simulink model "Suspension_system_nonlinear_dynamic_model"  (R2020a)
settings: Solver=FixedStepAuto  StartTime=0.0  StopTime=10  FixedStep=0.01  RelTol=1e-3
undefined symbols (not defined in the file): Ab1, Ab2, Agp, Ao1, Ao2, Apis, Ar, Arod, Av, b, Cdb1, Cdb2, Cdo1, Cdo2, Cdv1, Cdv2, Cf, Dpis, Dv1, Dv2, Fsp, k1, k2, l, Lg, mgp, Mpassm, mu, Pgasi, rho, slugs
libraries: simulink x9
settings Model: Creator=jmoyj  LastModifiedBy=jmoyj
settings DataIOCC: ReturnWorkspaceOutputs=off
settings DebuggingCC: ArithmeticOperatorsInVariantConditions=warning
settings SFSimCC: CustomCodeUndefinedFunction=UseInterfaceOnly

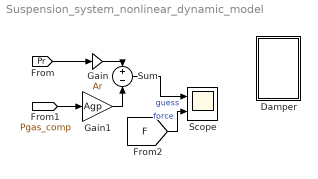
== system Suspension_system_nonlinear_dynamic_model ==
  Damper : Subsystem
  Gain : Gain  Gain=Ar
  Gain1 : Gain  Gain=Agp
  Scope : Scope  NumInputPorts=2
  Sum : Sum  Inputs=+-
  wires:
  [Pr] -> Gain/1
  [Pgas_comp] -> Gain1/1
  Gain/1 -> Sum/1
  Gain1/1 -> Sum/2
  Sum/1 -> Scope/1  "guess"
  [F] -> Scope/2  "force"

== system Suspension_system_nonlinear_dynamic_model/Damper ==
  Compression : Subsystem
  Final Values : Subsystem
  "Inputs_data " : Subsystem
  Rebound : Subsystem
  Scope10 : Scope
  Scope11 : Scope
  wires:
  "Inputs_data "/1(velocity) -> Scope11/1  "Velocity"
  "Inputs_data "/2(displacement) -> Scope10/1  "distance"

== system Suspension_system_nonlinear_dynamic_model/Damper/Compression ==
  " Q" : Subsystem
  CR : Subsystem
  CV : Subsystem
  Force : Subsystem
  Pgas and Pc : Subsystem
  Pr,Pc,Pv : Subsystem
  "Qb " : Subsystem
  Qlp : Subsystem
  "Qv " : Subsystem
  Scope : Scope  NumInputPorts=2
  Scope1 : Scope
  Sum : Sum  Inputs=|++
  "y " : Subsystem
  wires:
  [Pc_common] -> Sum/2, Scope/1
  [Pc_rebound] -> Sum/1, Scope/2
  Sum/1 -> Scope1/1

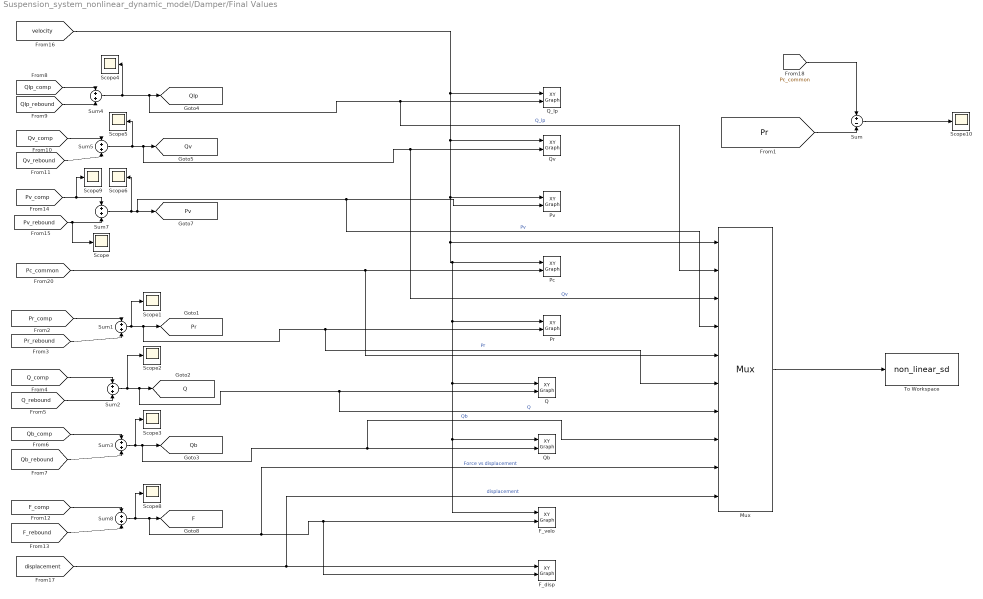
== system Suspension_system_nonlinear_dynamic_model/Damper/Final Values ==
  F_disp : simulink/Sinks/XY Graph  xmin=-1  xmax=+1  ymin=-20  ymax=30  st=-1
  F_velo : simulink/Sinks/XY Graph  xmin=-6  xmax=+6  ymin=-20  ymax=20  st=-1
  Mux : Mux  Inputs=10
  Pc : simulink/Sinks/XY Graph  xmin=-6  xmax=+6  ymin=20  ymax=30  st=-1
  Pr : simulink/Sinks/XY Graph  xmin=-6  xmax=+6  ymin=5  ymax=45  st=-1
  Pv : simulink/Sinks/XY Graph  xmin=-6  xmax=+6  ymin=12  ymax=40  st=-1
  Q : simulink/Sinks/XY Graph  xmin=-6  xmax=+6  ymin=0  ymax=5  st=-1
  Q_lp : simulink/Sinks/XY Graph  xmin=-6  xmax=6  ymin=0  ymax=0.005  st=-1
  Qb : simulink/Sinks/XY Graph  xmin=-6  xmax=+6  ymin=0  ymax=5  st=-1
  Qv : simulink/Sinks/XY Graph  xmin=-6  xmax=+6  ymin=0  ymax=1.5  st=-1
  Scope{,1..6,8..10} (10 alike) : Scope
  Sum : Sum  Inputs=+-
  Sum{1..5,7..8} (7 alike) : Sum
  To Workspace : ToWorkspace  VariableName=non_linear_sd  SaveFormat=Timeseries  SampleTime=-1
  tag scope: F=global, Pr=global, Pv=global, Q=global, Qb=global, Qlp=global, Qv=global
  wires:
  Sum1/1 -> Scope1/1, Mux/6, Pr/2, [Pr]  "Pr"
  [Pr_comp] -> Sum1/1
  [Pr_rebound] -> Sum1/2
  Sum2/1 -> Scope2/1, Mux/7, Q/2, [Q]  "Q"
  [Q_comp] -> Sum2/1
  [Q_rebound] -> Sum2/2
  Sum3/1 -> Scope3/1, Mux/8, Qb/2, [Qb]  "Qb"
  [Qb_comp] -> Sum3/1
  [Qb_rebound] -> Sum3/2
  Sum4/1 -> Scope4/1, Mux/2, Q_lp/2, [Qlp]  "Q_lp"
  [Qlp_comp] -> Sum4/1
  [Qlp_rebound] -> Sum4/2
  Sum5/1 -> Scope5/1, Mux/3, Qv/2, [Qv]  "Qv"
  [Qv_comp] -> Sum5/1
  [Qv_rebound] -> Sum5/2
  [Pv_rebound] -> Scope/1, Sum7/2
  Sum7/1 -> Scope6/1, Mux/4, Pv/2, [Pv]  "Pv"
  [Pv_comp] -> Scope9/1, Sum7/1
  Sum8/1 -> Scope8/1, Mux/9, F_disp/2, F_velo/2, [F]  "Force vs displacement"
  [F_comp] -> Sum8/1
  [F_rebound] -> Sum8/2
  [velocity] -> Mux/1, F_velo/1, Qb/1, Q/1, Pr/1, Pc/1, Pv/1, Qv/1, Q_lp/1
  [displacement] -> Mux/10, F_disp/1  "displacement"
  Mux/1 -> To Workspace/1
  [Pc_common] -> Sum/1
  [Pr] -> Sum/2
  Sum/1 -> Scope10/1
  [Pc_common] -> Mux/5, Pc/2

== system Suspension_system_nonlinear_dynamic_model/Damper/Inputs_data  ==
  Derivative : Derivative
  Derivative1 : Derivative
  Scope : Scope
  Scope1 : Scope
  Scope2 : Scope
  Sine Wave : Sin  Amplitude=0.499  Frequency=1.59*2*pi  Phase=-(pi/2)  SampleTime=0
  velocity : Outport  VectorParamsAs1DForOutWhenUnconnected=off
  displacement : Outport  Port=2  VectorParamsAs1DForOutWhenUnconnected=off
  tag scope: acceleration=global, displacement=global, velocity=global
  wires:
  Derivative1/1 -> [acceleration], Scope2/1
  Derivative/1 -> velocity/1, Scope1/1, [velocity], Derivative1/1
  Sine Wave/1 -> Derivative/1, displacement/1, Scope/1, [displacement]

== system Suspension_system_nonlinear_dynamic_model/Damper/Rebound ==
  " Q" : Subsystem
  Force Model : Subsystem
  Pc,Pr,Pv : Subsystem
  Pgas and Pc : Subsystem
  "Qb " : Subsystem
  Qlp : Subsystem
  "Qv " : Subsystem
  RC : Subsystem
  RV : Subsystem
  "y " : Subsystem

== system Suspension_system_nonlinear_dynamic_model/Damper/Compression/ Q ==
  Constant : Constant  Value=Ar
  Constant1 : Constant  Value=0
  Product : Product
  Scope : Scope
  Sign : Signum
  Switch : Switch  Criteria=u2 > Threshold
  tag scope: Q_comp=global
  wires:
  Constant/1 -> Product/2
  [velocity] -> Sign/1, Product/1
  Product/1 -> Switch/1
  Sign/1 -> Switch/2
  Constant1/1 -> Switch/3
  Switch/1 -> Scope/1, [Q_comp]

== system Suspension_system_nonlinear_dynamic_model/Damper/Compression/CR ==
  Constant : Constant  Value=rho
  Constant1 : Constant  Value=2
  Constant2 : Constant  Value=slugs
  Constant3 : Constant  Value=Ab1
  Constant4 : Constant  Value=Cdb1
  Delay : Delay  DelayLength=0  InitialCondition=0.02
  Product : Product
  Product1 : Product  Inputs=3
  Product2 : Product  Inputs=*/
  Product3 : Product
  Scope1 : Scope
  Scope2 : Scope
  Square : Math  Operator=square  SignedPower=on  SaturateOnIntegerOverflow=on
  Square1 : Math  Operator=square  SignedPower=on  SaturateOnIntegerOverflow=on
  tag scope: CR=global
  wires:
  Product1/1 -> Product2/2
  Product/1 -> Product2/1
  Square1/1 -> Product1/3
  Constant/1 -> Product/1
  Constant2/1 -> Product1/2
  Constant4/1 -> Product3/2
  Constant1/1 -> Product1/1
  Square/1 -> Product/2
  [Qb_comp] -> Scope1/1, Square/1
  Product3/1 -> Square1/1
  Constant3/1 -> Product3/1
  Product2/1 -> Scope2/1, Delay/1
  Delay/1 -> [CR]

== system Suspension_system_nonlinear_dynamic_model/Damper/Compression/CV ==
  Constant : Constant  Value=rho
  Constant1 : Constant  Value=2
  Constant2 : Constant  Value=slugs
  Constant3 : Constant  Value=Ao1
  Constant4 : Constant  Value=Cdo1
  Delay : Delay  DelayLength=0  InitialCondition=0.16
  Product : Product
  Product1 : Product  Inputs=3
  Product2 : Product  Inputs=*/
  Product3 : Product
  Scope{,1..3} (4 alike) : Scope
  Square : Math  Operator=square  SignedPower=on  SaturateOnIntegerOverflow=on
  Square1 : Math  Operator=square  SignedPower=on  SaturateOnIntegerOverflow=on
  tag scope: CV=global
  wires:
  Product1/1 -> Product2/2, Scope2/1
  Product/1 -> Product2/1
  Square1/1 -> Product1/3
  Constant/1 -> Product/1
  Constant2/1 -> Product1/2
  Constant4/1 -> Product3/2
  Constant1/1 -> Product1/1
  Square/1 -> Product/2
  [Qv_comp] -> Scope/1, Square/1
  Product3/1 -> Square1/1
  Constant3/1 -> Product3/1
  Delay/1 -> Scope3/1, [CV]
  Product2/1 -> Scope1/1, Delay/1

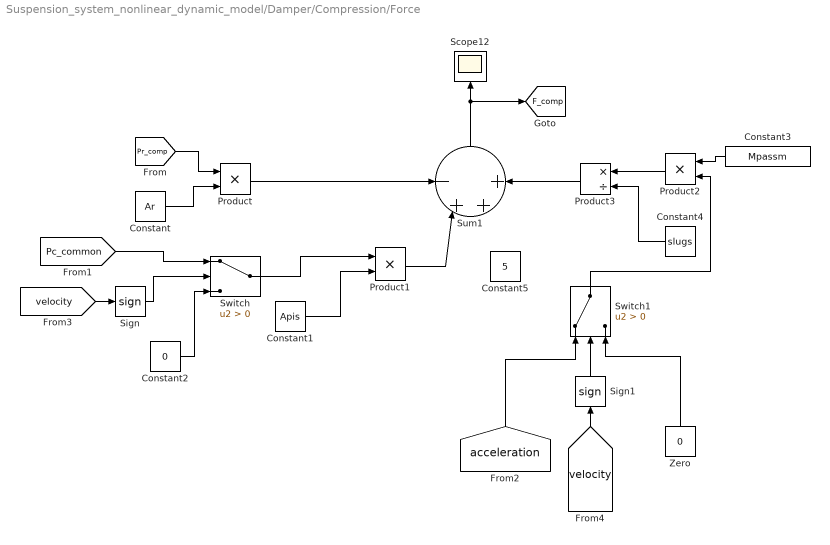
== system Suspension_system_nonlinear_dynamic_model/Damper/Compression/Force ==
  Constant : Constant  Value=Ar
  Constant1 : Constant  Value=Apis
  Constant2 : Constant  Value=0
  Constant3 : Constant  Value=Mpassm
  Constant4 : Constant  Value=slugs
  Constant5 : Constant  Value=5
  Product : Product
  Product1 : Product
  Product2 : Product
  Product3 : Product  Inputs=*/
  Scope12 : Scope
  Sign : Signum
  Sign1 : Signum
  Sum1 : Sum  Inputs=-+++
  Switch : Switch  Criteria=u2 > Threshold
  Switch1 : Switch  Criteria=u2 > Threshold
  Zero : Constant  Value=0  OutDataTypeStr=Inherit: Inherit via back propagation
  tag scope: F_comp=global
  wires:
  Constant1/1 -> Product1/2
  Product2/1 -> Product3/1
  Sum1/1 -> [F_comp], Scope12/1
  Constant/1 -> Product/2
  Product1/1 -> Sum1/2
  Switch1/1 -> Product2/2
  Constant3/1 -> Product2/1
  Product/1 -> Sum1/1
  [Pr_comp] -> Product/1
  Constant4/1 -> Product3/2
  Product3/1 -> Sum1/4
  [Pc_common] -> Switch/1
  Switch/1 -> Product1/1
  [velocity] -> Sign/1
  Constant2/1 -> Switch/3
  Sign/1 -> Switch/2
  [acceleration] -> Switch1/1
  Sign1/1 -> Switch1/2
  [velocity] -> Sign1/1
  Zero/1 -> Switch1/3

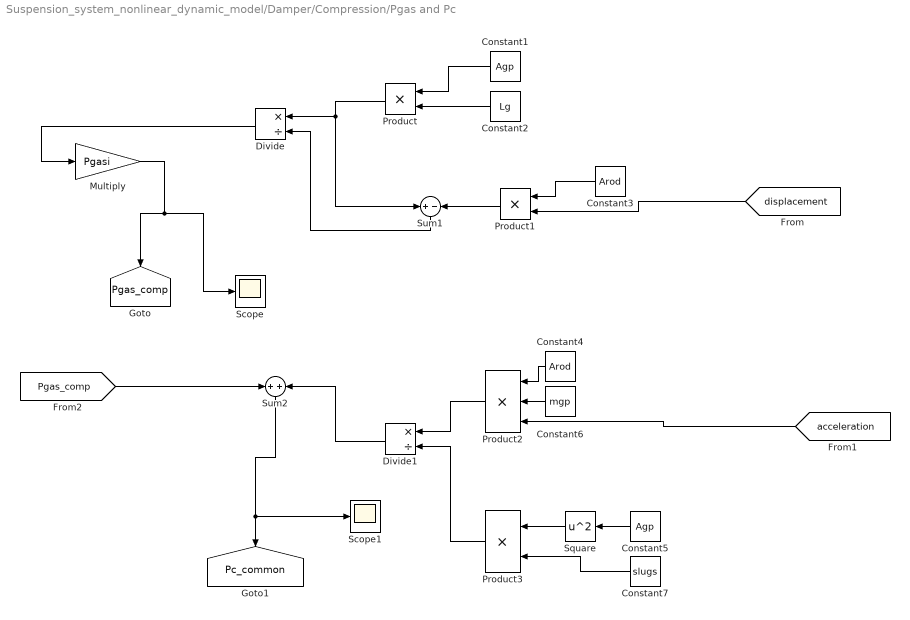
== system Suspension_system_nonlinear_dynamic_model/Damper/Compression/Pgas and Pc ==
  Constant1 : Constant  Value=Agp
  Constant2 : Constant  Value=Lg
  Constant3 : Constant  Value=Arod
  Constant4 : Constant  Value=Arod
  Constant5 : Constant  Value=Agp
  Constant6 : Constant  Value=mgp
  Constant7 : Constant  Value=slugs
  Divide : Product  Inputs=*/
  Divide1 : Product  Inputs=*/
  Multiply : Gain  Gain=Pgasi
  Product : Product
  Product1 : Product
  Product2 : Product  Inputs=3
  Product3 : Product
  Scope : Scope
  Scope1 : Scope
  Square : Math  Operator=square  SignedPower=on  SaturateOnIntegerOverflow=on
  Sum1 : Sum  Inputs=+-
  Sum2 : Sum
  tag scope: Pc_common=global, Pgas_comp=global
  wires:
  Constant6/1 -> Product2/2
  Constant3/1 -> Product1/1
  Constant4/1 -> Product2/1
  Constant5/1 -> Square/1
  Product2/1 -> Divide1/1
  Product/1 -> Sum1/1, Divide/1
  Multiply/1 -> [Pgas_comp], Scope/1
  Constant2/1 -> Product/2
  Product1/1 -> Sum1/2
  Divide1/1 -> Sum2/2
  Constant1/1 -> Product/1
  Sum1/1 -> Divide/2
  Divide/1 -> Multiply/1
  Constant7/1 -> Product3/2
  Product3/1 -> Divide1/2
  Square/1 -> Product3/1
  [Pgas_comp] -> Sum2/1
  Sum2/1 -> Scope1/1, [Pc_common]
  [acceleration] -> Product2/3
  [displacement] -> Product1/2

== system Suspension_system_nonlinear_dynamic_model/Damper/Compression/Pr,Pc,Pv ==
  Constant : Constant  Value=0
  Delay : Delay  DelayLength=0  InitialCondition=26.24
  Delay1 : Delay  DelayLength=0  InitialCondition=26.07
  Sign : Signum
  Sum : Sum  Inputs=+-
  Sum1 : Sum  Inputs=-+
  Sum2 : Sum
  Switch : Switch  Criteria=u2 > Threshold
  tag scope: Pr_comp=global, Pv_comp=global, VR=global
  wires:
  Switch/1 -> Sum1/2
  Sum/1 -> [VR]
  [VR] -> Sum2/1
  Sum1/1 -> Delay1/1
  [CR] -> Sum1/1
  [CR] -> Sum/1
  [velocity] -> Sign/1
  [CV] -> Sum/2
  Sum2/1 -> Delay/1
  [Pc_common] -> Switch/1
  Constant/1 -> Switch/3
  Sign/1 -> Switch/2
  [Pr_comp] -> Sum2/2
  Delay/1 -> [Pv_comp]
  Delay1/1 -> [Pr_comp]

== system Suspension_system_nonlinear_dynamic_model/Damper/Compression/Qb  ==
  Complex to Real-Imag : ComplexToRealImag  Output=Real
  Delay1 : Delay  DelayLength=0  InitialCondition=0.35
  Scope : Scope
  Scope1 : Scope
  Sum : Sum  Inputs=+--
  tag scope: Qb_comp=global
  wires:
  [Qv_comp] -> Scope1/1, Sum/2
  [Qlp_comp] -> Sum/3
  [Q_comp] -> Sum/1
  Sum/1 -> Scope/1, Complex to Real-Imag/1
  Delay1/1 -> [Qb_comp]
  Complex to Real-Imag/1 -> Delay1/1

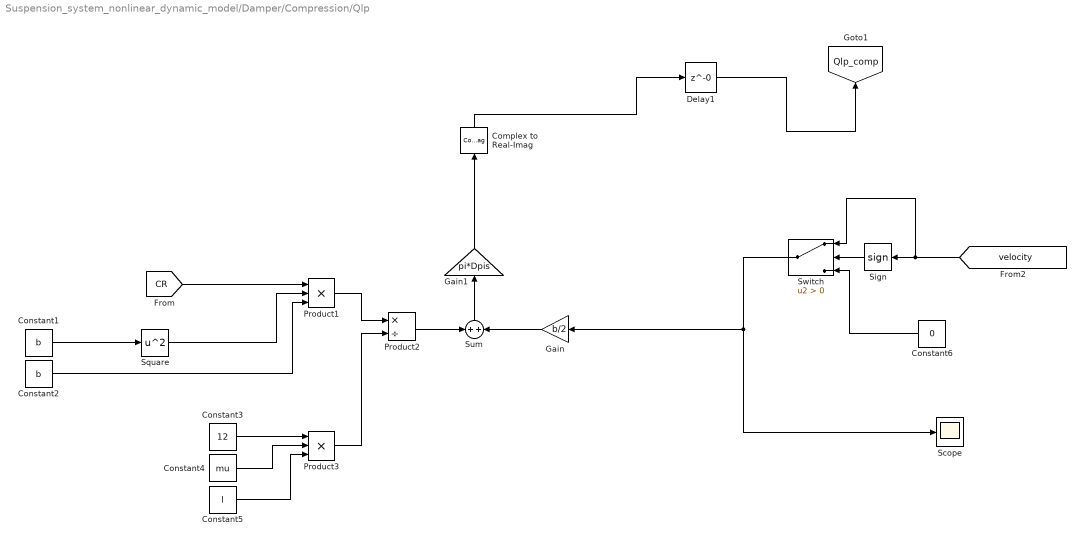
== system Suspension_system_nonlinear_dynamic_model/Damper/Compression/Qlp ==
  Complex to Real-Imag : ComplexToRealImag  Output=Real
  Constant1 : Constant  Value=b
  Constant2 : Constant  Value=b
  Constant3 : Constant  Value=12
  Constant4 : Constant  Value=mu
  Constant5 : Constant  Value=l
  Constant6 : Constant  Value=0
  Delay1 : Delay  DelayLength=0  InitialCondition=0.0025
  Gain : Gain  Gain=b/2
  Gain1 : Gain  Gain=pi*Dpis
  Product1 : Product  Inputs=3
  Product2 : Product  Inputs=*/
  Product3 : Product  Inputs=3
  Scope : Scope
  Sign : Signum
  Square : Math  Operator=square  SignedPower=on  SaturateOnIntegerOverflow=on
  Sum : Sum
  Switch : Switch  Criteria=u2 > Threshold
  tag scope: Qlp_comp=global
  wires:
  Product3/1 -> Product2/2
  Constant1/1 -> Square/1
  Constant3/1 -> Product3/1
  Product1/1 -> Product2/1
  Square/1 -> Product1/2
  Switch/1 -> Gain/1, Scope/1
  [CR] -> Product1/1
  Constant2/1 -> Product1/3
  Gain/1 -> Sum/2
  Constant4/1 -> Product3/2
  Sum/1 -> Gain1/1
  Constant5/1 -> Product3/3
  Product2/1 -> Sum/1
  [velocity] -> Switch/1, Sign/1
  Gain1/1 -> Complex to Real-Imag/1
  Delay1/1 -> [Qlp_comp]
  Complex to Real-Imag/1 -> Delay1/1
  Sign/1 -> Switch/2
  Constant6/1 -> Switch/3

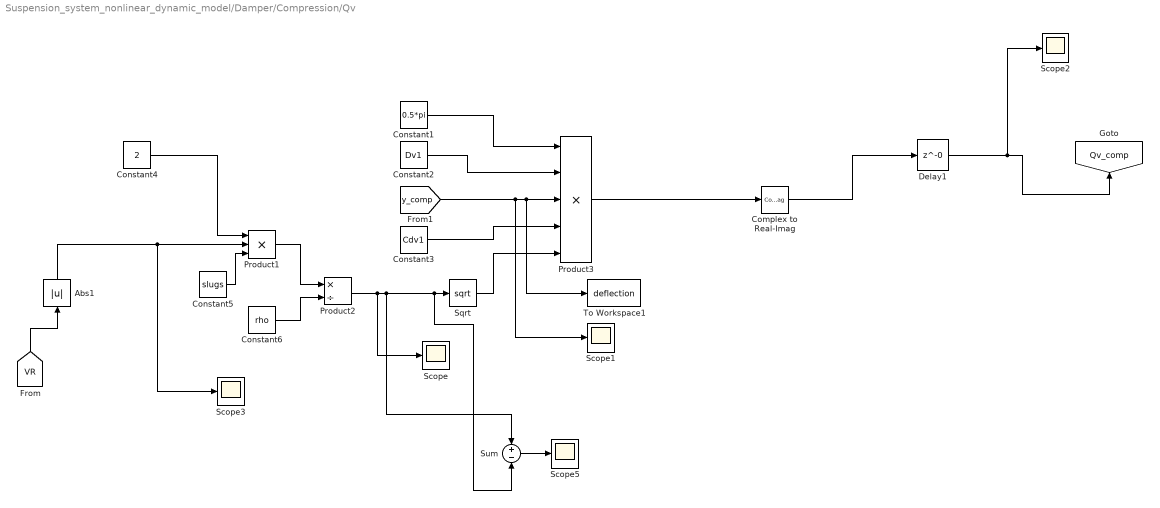
== system Suspension_system_nonlinear_dynamic_model/Damper/Compression/Qv  ==
  Abs1 : Abs
  Complex to Real-Imag : ComplexToRealImag  Output=Real
  Constant1 : Constant  Value=0.5*pi
  Constant2 : Constant  Value=Dv1
  Constant3 : Constant  Value=Cdv1
  Constant4 : Constant  Value=2
  Constant5 : Constant  Value=slugs
  Constant6 : Constant  Value=rho
  Delay1 : Delay  DelayLength=0  InitialCondition=0.08
  Product1 : Product  Inputs=3
  Product2 : Product  Inputs=*/
  Product3 : Product  Inputs=5
  Scope{,1..3,5} (5 alike) : Scope
  Sqrt : Sqrt  SaturateOnIntegerOverflow=on
  Sum : Sum  Inputs=+-
  To Workspace1 : ToWorkspace  VariableName=deflection  SaveFormat=Timeseries  SampleTime=-1
  tag scope: Qv_comp=global
  wires:
  Constant6/1 -> Product2/2
  [y_comp] -> To Workspace1/1, Product3/3, Scope1/1
  Constant2/1 -> Product3/2
  Constant3/1 -> Product3/4
  Product1/1 -> Product2/1
  Sqrt/1 -> Product3/5
  Constant1/1 -> Product3/1
  Constant4/1 -> Product1/1
  Constant5/1 -> Product1/3
  Product2/1 -> Scope/1, Sum/2, Sqrt/1, Sum/1
  Product3/1 -> Complex to Real-Imag/1
  Delay1/1 -> Scope2/1, [Qv_comp]
  Complex to Real-Imag/1 -> Delay1/1
  [VR] -> Abs1/1
  Abs1/1 -> Scope3/1, Product1/2
  Sum/1 -> Scope5/1

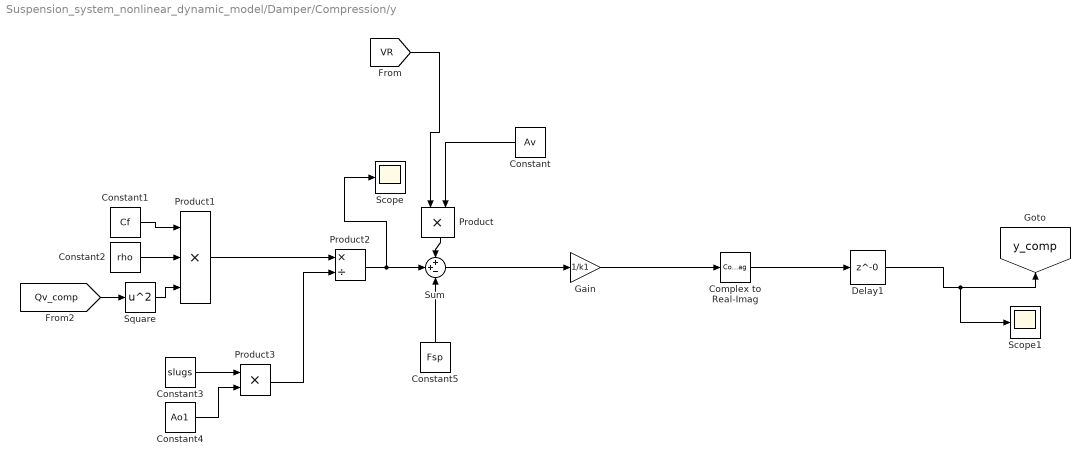
== system Suspension_system_nonlinear_dynamic_model/Damper/Compression/y  ==
  Complex to Real-Imag : ComplexToRealImag  Output=Real
  Constant : Constant  Value=Av
  Constant1 : Constant  Value=Cf
  Constant2 : Constant  Value=rho
  Constant3 : Constant  Value=slugs
  Constant4 : Constant  Value=Ao1
  Constant5 : Constant  Value=Fsp
  Delay1 : Delay  DelayLength=0  InitialCondition=0.0005
  Gain : Gain  Gain=1/k1
  Product : Product
  Product1 : Product  Inputs=3
  Product2 : Product  Inputs=*/
  Product3 : Product  Inputs=**
  Scope : Scope
  Scope1 : Scope
  Square : Math  Operator=square  SignedPower=on  SaturateOnIntegerOverflow=on
  Sum : Sum  Inputs=++-
  tag scope: y_comp=global
  wires:
  Product2/1 -> Scope/1, Sum/2
  Constant2/1 -> Product1/2
  Square/1 -> Product1/3
  Constant3/1 -> Product3/1
  Sum/1 -> Gain/1
  Constant1/1 -> Product1/1
  Constant4/1 -> Product3/2
  [Qv_comp] -> Square/1
  Product1/1 -> Product2/1
  Product/1 -> Sum/1
  Constant/1 -> Product/2
  Product3/1 -> Product2/2
  Constant5/1 -> Sum/3
  Gain/1 -> Complex to Real-Imag/1
  Complex to Real-Imag/1 -> Delay1/1
  Delay1/1 -> Scope1/1, [y_comp]
  [VR] -> Product/1

== system Suspension_system_nonlinear_dynamic_model/Damper/Rebound/ Q ==
  Abs : Abs
  Constant : Constant  Value=Ar
  Constant1 : Constant  Value=0
  Product : Product
  Scope : Scope
  Sign : Signum
  Switch : Switch  Criteria=u2 > Threshold
  tag scope: Q_rebound=global
  wires:
  Constant/1 -> Product/2
  [velocity] -> Sign/1, Product/1
  Sign/1 -> Switch/2
  Switch/1 -> Scope/1, [Q_rebound]
  Constant1/1 -> Switch/1
  Product/1 -> Abs/1
  Abs/1 -> Switch/3

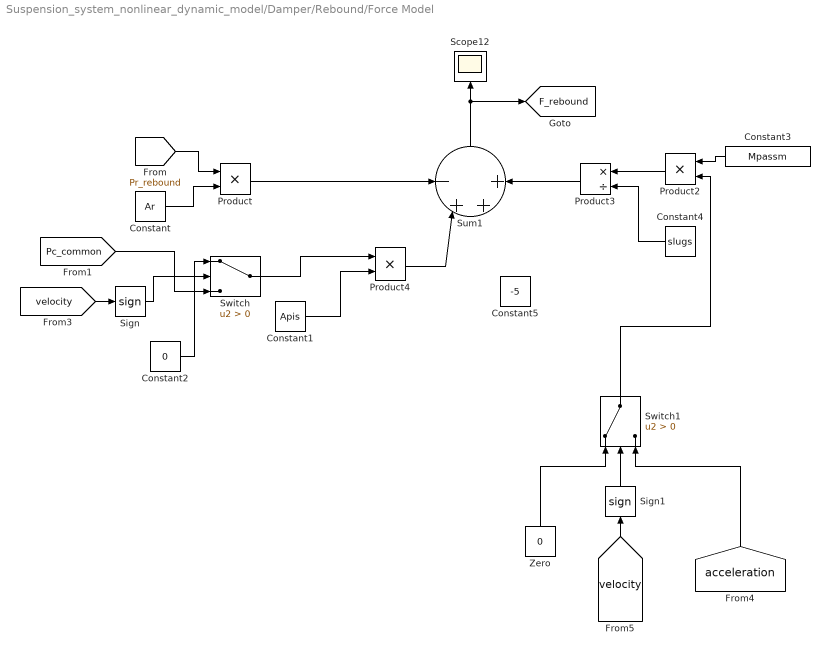
== system Suspension_system_nonlinear_dynamic_model/Damper/Rebound/Force Model ==
  Constant : Constant  Value=Ar
  Constant1 : Constant  Value=Apis
  Constant2 : Constant  Value=0
  Constant3 : Constant  Value=Mpassm
  Constant4 : Constant  Value=slugs
  Constant5 : Constant  Value=-5
  Product : Product
  Product2 : Product
  Product3 : Product  Inputs=*/
  Product4 : Product
  Scope12 : Scope
  Sign : Signum
  Sign1 : Signum
  Sum1 : Sum  Inputs=-+++
  Switch : Switch  Criteria=u2 > Threshold
  Switch1 : Switch  Criteria=u2 > Threshold
  Zero : Constant  Value=0  OutDataTypeStr=Inherit: Inherit via back propagation
  tag scope: F_rebound=global
  wires:
  Product2/1 -> Product3/1
  Sum1/1 -> [F_rebound], Scope12/1
  Constant/1 -> Product/2
  Switch1/1 -> Product2/2
  Constant3/1 -> Product2/1
  Product/1 -> Sum1/1
  [Pr_rebound] -> Product/1
  Constant4/1 -> Product3/2
  Product3/1 -> Sum1/4
  Constant1/1 -> Product4/2
  Product4/1 -> Sum1/2
  Switch/1 -> Product4/1
  Sign/1 -> Switch/2
  [velocity] -> Sign/1
  Constant2/1 -> Switch/1
  [Pc_common] -> Switch/3
  Sign1/1 -> Switch1/2
  [velocity] -> Sign1/1
  Zero/1 -> Switch1/1
  [acceleration] -> Switch1/3

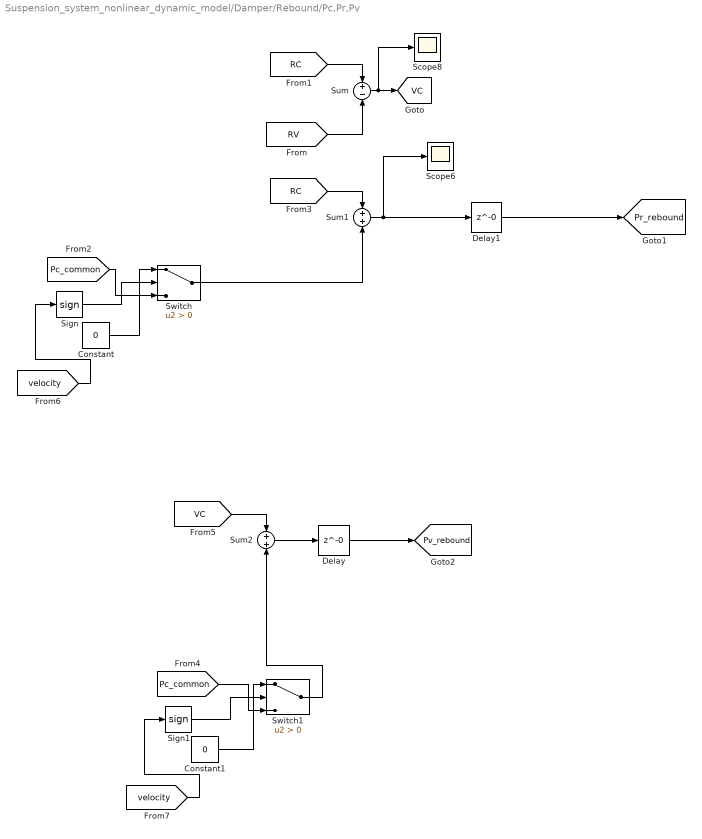
== system Suspension_system_nonlinear_dynamic_model/Damper/Rebound/Pc,Pr,Pv ==
  Constant : Constant  Value=0
  Constant1 : Constant  Value=0
  Delay : Delay  DelayLength=0  InitialCondition=32.9
  Delay1 : Delay  DelayLength=0  InitialCondition=32.1
  Scope6 : Scope
  Scope8 : Scope
  Sign : Signum
  Sign1 : Signum
  Sum : Sum  Inputs=+-
  Sum1 : Sum
  Sum2 : Sum
  Switch : Switch  Criteria=u2 > Threshold
  Switch1 : Switch  Criteria=u2 > Threshold
  tag scope: Pr_rebound=global, Pv_rebound=global, VC=global
  wires:
  [velocity] -> Sign/1
  [RC] -> Sum1/1
  Sum1/1 -> Scope6/1, Delay1/1
  Sum/1 -> Scope8/1, [VC]
  Switch/1 -> Sum1/2
  [RC] -> Sum/1
  Constant/1 -> Switch/1
  Sign/1 -> Switch/2
  [Pc_common] -> Switch/3
  [RV] -> Sum/2
  Constant1/1 -> Switch1/1
  [VC] -> Sum2/1
  Switch1/1 -> Sum2/2
  Sum2/1 -> Delay/1
  [Pc_common] -> Switch1/3
  [velocity] -> Sign1/1
  Sign1/1 -> Switch1/2
  Delay/1 -> [Pv_rebound]
  Delay1/1 -> [Pr_rebound]

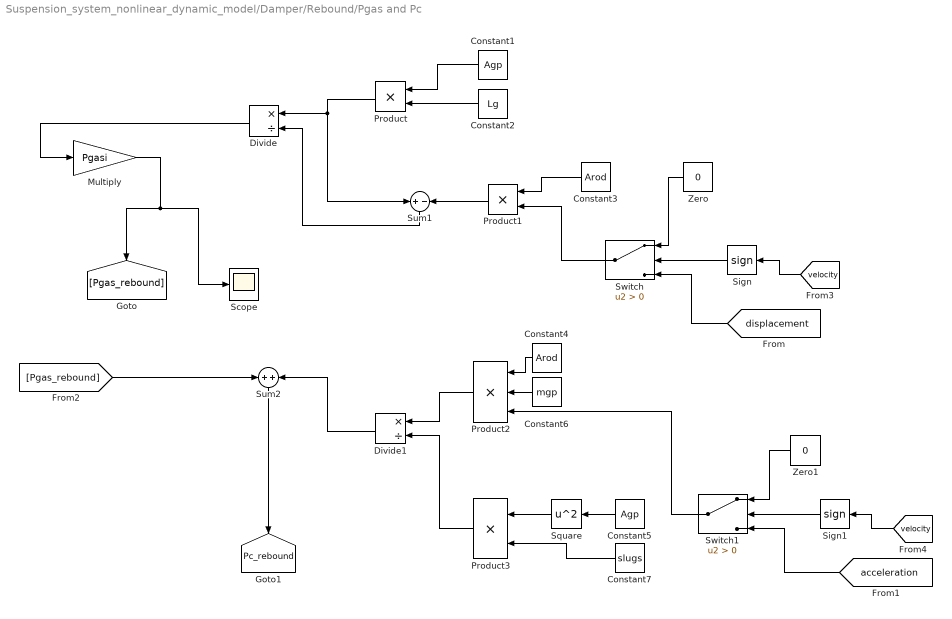
== system Suspension_system_nonlinear_dynamic_model/Damper/Rebound/Pgas and Pc ==
  Constant1 : Constant  Value=Agp
  Constant2 : Constant  Value=Lg
  Constant3 : Constant  Value=Arod
  Constant4 : Constant  Value=Arod
  Constant5 : Constant  Value=Agp
  Constant6 : Constant  Value=mgp
  Constant7 : Constant  Value=slugs
  Divide : Product  Inputs=*/
  Divide1 : Product  Inputs=*/
  Multiply : Gain  Gain=Pgasi
  Product : Product
  Product1 : Product
  Product2 : Product  Inputs=3
  Product3 : Product
  Scope : Scope
  Sign : Signum
  Sign1 : Signum
  Square : Math  Operator=square  SignedPower=on  SaturateOnIntegerOverflow=on
  Sum1 : Sum  Inputs=+-
  Sum2 : Sum
  Switch : Switch  Criteria=u2 > Threshold
  Switch1 : Switch  Criteria=u2 > Threshold
  Zero : Constant  Value=0  OutDataTypeStr=Inherit: Inherit via back propagation
  Zero1 : Constant  Value=0  OutDataTypeStr=Inherit: Inherit via back propagation
  tag scope: Pc_rebound=global
  wires:
  Constant6/1 -> Product2/2
  Constant3/1 -> Product1/1
  Constant4/1 -> Product2/1
  Constant5/1 -> Square/1
  Product2/1 -> Divide1/1
  Product/1 -> Sum1/1, Divide/1
  Multiply/1 -> [Pgas_rebound], Scope/1
  Constant2/1 -> Product/2
  Product1/1 -> Sum1/2
  Divide1/1 -> Sum2/2
  Constant1/1 -> Product/1
  Sum1/1 -> Divide/2
  Divide/1 -> Multiply/1
  Constant7/1 -> Product3/2
  Product3/1 -> Divide1/2
  Square/1 -> Product3/1
  [Pgas_rebound] -> Sum2/1
  Sum2/1 -> [Pc_rebound]
  Switch/1 -> Product1/2
  [velocity] -> Sign/1
  Sign/1 -> Switch/2
  Sign1/1 -> Switch1/2
  [velocity] -> Sign1/1
  Switch1/1 -> Product2/3
  [displacement] -> Switch/3
  Zero/1 -> Switch/1
  Zero1/1 -> Switch1/1
  [acceleration] -> Switch1/3

== system Suspension_system_nonlinear_dynamic_model/Damper/Rebound/Qb  ==
  Complex to Real-Imag : ComplexToRealImag  Output=Real
  Delay1 : Delay  DelayLength=0  InitialCondition=0.5
  Scope : Scope
  Scope1 : Scope
  Sum : Sum  Inputs=+--
  tag scope: Qb_rebound=global
  wires:
  [Qv_rebound] -> Scope1/1, Sum/2
  [Qlp_rebound] -> Sum/3
  [Q_rebound] -> Sum/1
  Sum/1 -> Scope/1, Complex to Real-Imag/1
  Delay1/1 -> [Qb_rebound]
  Complex to Real-Imag/1 -> Delay1/1

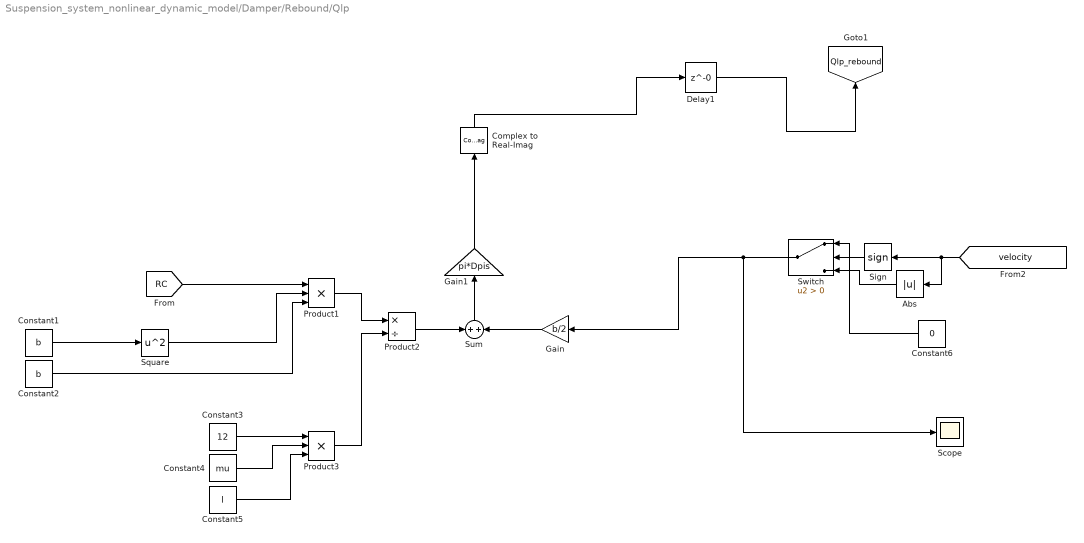
== system Suspension_system_nonlinear_dynamic_model/Damper/Rebound/Qlp ==
  Abs : Abs
  Complex to Real-Imag : ComplexToRealImag  Output=Real
  Constant1 : Constant  Value=b
  Constant2 : Constant  Value=b
  Constant3 : Constant  Value=12
  Constant4 : Constant  Value=mu
  Constant5 : Constant  Value=l
  Constant6 : Constant  Value=0
  Delay1 : Delay  DelayLength=0  InitialCondition=0.005
  Gain : Gain  Gain=b/2
  Gain1 : Gain  Gain=pi*Dpis
  Product1 : Product  Inputs=3
  Product2 : Product  Inputs=*/
  Product3 : Product  Inputs=3
  Scope : Scope
  Sign : Signum
  Square : Math  Operator=square  SignedPower=on  SaturateOnIntegerOverflow=on
  Sum : Sum
  Switch : Switch  Criteria=u2 > Threshold
  tag scope: Qlp_rebound=global
  wires:
  Product3/1 -> Product2/2
  Constant1/1 -> Square/1
  Constant3/1 -> Product3/1
  Product1/1 -> Product2/1
  Square/1 -> Product1/2
  [RC] -> Product1/1
  Constant2/1 -> Product1/3
  Gain/1 -> Sum/2
  Constant4/1 -> Product3/2
  Sum/1 -> Gain1/1
  Constant5/1 -> Product3/3
  Product2/1 -> Sum/1
  [velocity] -> Abs/1, Sign/1
  Switch/1 -> Gain/1, Scope/1
  Gain1/1 -> Complex to Real-Imag/1
  Delay1/1 -> [Qlp_rebound]
  Complex to Real-Imag/1 -> Delay1/1
  Sign/1 -> Switch/2
  Constant6/1 -> Switch/1
  Abs/1 -> Switch/3

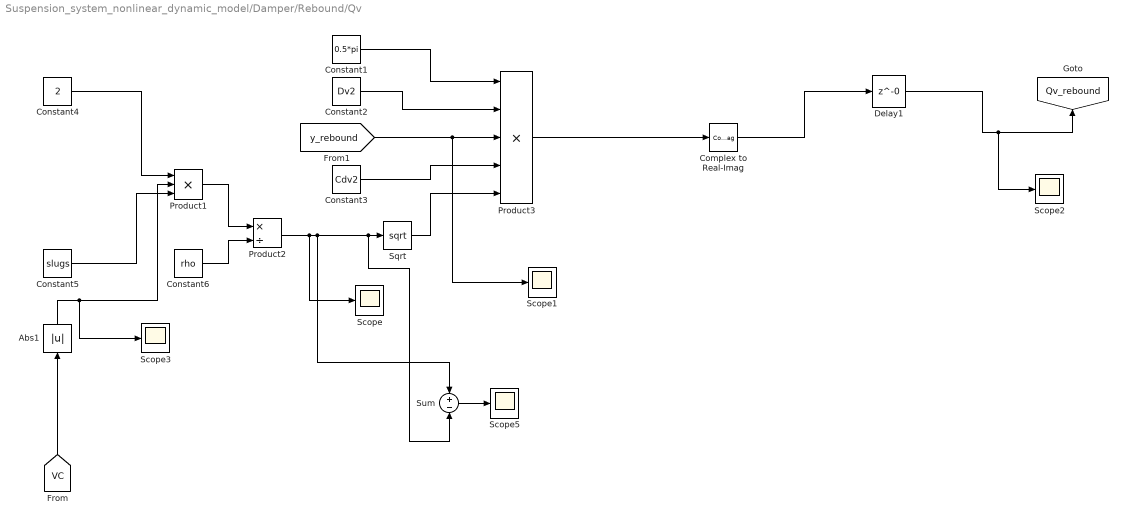
== system Suspension_system_nonlinear_dynamic_model/Damper/Rebound/Qv  ==
  Abs1 : Abs
  Complex to Real-Imag : ComplexToRealImag  Output=Real
  Constant1 : Constant  Value=0.5*pi
  Constant2 : Constant  Value=Dv2
  Constant3 : Constant  Value=Cdv2
  Constant4 : Constant  Value=2
  Constant5 : Constant  Value=slugs
  Constant6 : Constant  Value=rho
  Delay1 : Delay  DelayLength=0  InitialCondition=0.5
  Product1 : Product  Inputs=3
  Product2 : Product  Inputs=*/
  Product3 : Product  Inputs=5
  Scope{,1..3,5} (5 alike) : Scope
  Sqrt : Sqrt  SaturateOnIntegerOverflow=on
  Sum : Sum  Inputs=+-
  tag scope: Qv_rebound=global
  wires:
  Constant6/1 -> Product2/2
  [y_rebound] -> Product3/3, Scope1/1
  Constant2/1 -> Product3/2
  Constant3/1 -> Product3/4
  Product1/1 -> Product2/1
  Sqrt/1 -> Product3/5
  Constant1/1 -> Product3/1
  Constant4/1 -> Product1/1
  Constant5/1 -> Product1/3
  Product2/1 -> Scope/1, Sum/2, Sqrt/1, Sum/1
  Product3/1 -> Complex to Real-Imag/1
  Delay1/1 -> Scope2/1, [Qv_rebound]
  Complex to Real-Imag/1 -> Delay1/1
  [VC] -> Abs1/1
  Abs1/1 -> Scope3/1, Product1/2
  Sum/1 -> Scope5/1

== system Suspension_system_nonlinear_dynamic_model/Damper/Rebound/RC ==
  Constant : Constant  Value=rho
  Constant1 : Constant  Value=2
  Constant2 : Constant  Value=slugs
  Constant3 : Constant  Value=Ab2
  Constant4 : Constant  Value=Cdb2
  Product : Product
  Product1 : Product  Inputs=3
  Product2 : Product  Inputs=*/
  Product3 : Product
  Scope1 : Scope
  Scope2 : Scope
  Square : Math  Operator=square  SignedPower=on  SaturateOnIntegerOverflow=on
  Square1 : Math  Operator=square  SignedPower=on  SaturateOnIntegerOverflow=on
  tag scope: RC=global
  wires:
  Product1/1 -> Product2/2
  Product/1 -> Product2/1
  Square1/1 -> Product1/3
  Constant/1 -> Product/1
  Constant2/1 -> Product1/2
  Constant4/1 -> Product3/2
  Constant1/1 -> Product1/1
  Square/1 -> Product/2
  [Qb_rebound] -> Scope1/1, Square/1
  Product3/1 -> Square1/1
  Constant3/1 -> Product3/1
  Product2/1 -> Scope2/1, [RC]

== system Suspension_system_nonlinear_dynamic_model/Damper/Rebound/RV ==
  Constant : Constant  Value=rho
  Constant1 : Constant  Value=2
  Constant2 : Constant  Value=slugs
  Constant3 : Constant  Value=Ao2
  Constant4 : Constant  Value=Cdo2
  Delay : Delay  DelayLength=0  InitialCondition=0.8
  Product : Product
  Product1 : Product  Inputs=3
  Product2 : Product  Inputs=*/
  Product3 : Product
  Scope : Scope
  Scope2 : Scope
  Square : Math  Operator=square  SignedPower=on  SaturateOnIntegerOverflow=on
  Square1 : Math  Operator=square  SignedPower=on  SaturateOnIntegerOverflow=on
  tag scope: RV=global
  wires:
  Product1/1 -> Product2/2, Scope2/1
  Product/1 -> Product2/1
  Square1/1 -> Product1/3
  Constant/1 -> Product/1
  Constant2/1 -> Product1/2
  Constant4/1 -> Product3/2
  Constant1/1 -> Product1/1
  Square/1 -> Product/2
  [Qv_rebound] -> Scope/1, Square/1
  Product3/1 -> Square1/1
  Constant3/1 -> Product3/1
  Product2/1 -> Delay/1
  Delay/1 -> [RV]

== system Suspension_system_nonlinear_dynamic_model/Damper/Rebound/y  ==
  Complex to Real-Imag : ComplexToRealImag  Output=Real
  Constant : Constant  Value=Av
  Constant1 : Constant  Value=Cf
  Constant2 : Constant  Value=rho
  Constant3 : Constant  Value=slugs
  Constant4 : Constant  Value=Ao2
  Constant5 : Constant  Value=Fsp
  Delay2 : Delay  DelayLength=0  InitialCondition=0.002
  Gain : Gain  Gain=1/k2
  Product : Product
  Product1 : Product  Inputs=3
  Product2 : Product  Inputs=*/
  Product3 : Product  Inputs=**
  Scope : Scope
  Scope1 : Scope
  Square : Math  Operator=square  SignedPower=on  SaturateOnIntegerOverflow=on
  Sum : Sum  Inputs=++-
  tag scope: y_rebound=global
  wires:
  Product2/1 -> Scope/1, Sum/2
  Constant2/1 -> Product1/2
  Square/1 -> Product1/3
  Constant3/1 -> Product3/1
  Sum/1 -> Gain/1
  Constant1/1 -> Product1/1
  Constant4/1 -> Product3/2
  [Qv_rebound] -> Square/1
  Product1/1 -> Product2/1
  Product/1 -> Sum/1
  Constant/1 -> Product/2
  Product3/1 -> Product2/2
  Constant5/1 -> Sum/3
  Gain/1 -> Complex to Real-Imag/1
  Complex to Real-Imag/1 -> Delay2/1
  Delay2/1 -> Scope1/1, [y_rebound]
  [VC] -> Product/1
